simulink model "Ballbeam2020a"  (R2020a)
settings: Solver=VariableStepAuto  StartTime=0.0  StopTime=inf  RelTol=1e-3
values from neighbouring files (symbols this model uses):
  d = 0.03    [ballbeam.m]
  Den = [1 0 0]    [ballbeam.m]
  Kd = 40    [ballbeam.m]
  Kp = 15    [ballbeam.m]
  L = 1.0    (= 1)    [ballbeam.m]
  Num = [-K]    [ballbeam.m]
  R = 5    [ballbeam.m]
libraries: aerolibconvert2 x1, simulink x1, vrlib x1
settings Model: Creator=asus  LastModifiedBy=asus

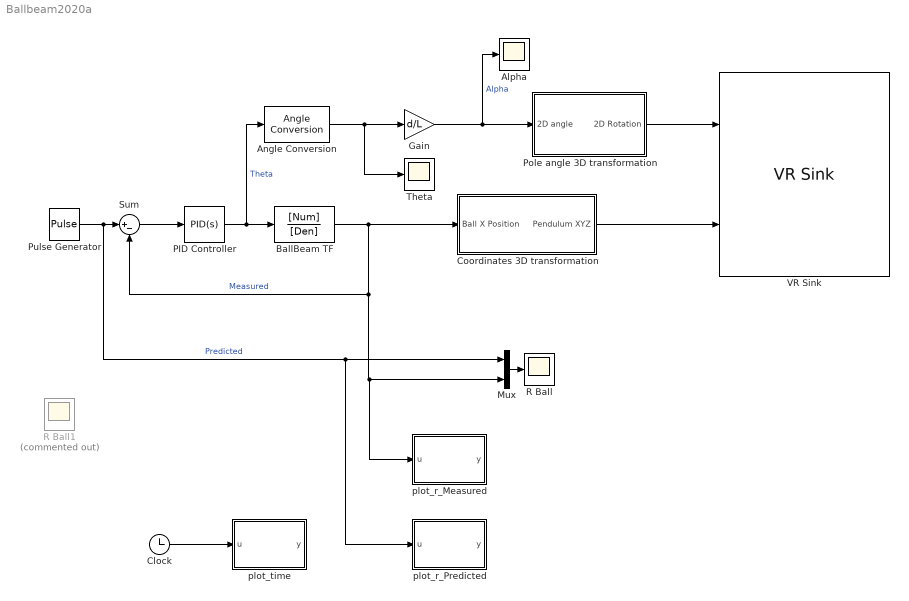
== system Ballbeam2020a ==
  "Alpha " : Scope
  Angle Conversion : aerolibconvert2/Angle Conversion  IU=deg  OU=rad
  BallBeam TF : TransferFcn  Numerator=[Num]  Denominator=[Den]
  Clock : Clock
  Coordinates 3D transformation : Subsystem
  Gain : Gain  Gain=d/L
  Mux : Mux  Inputs=2
  PID Controller : simulink/Continuous/PID Controller  Controller=PID  Form=Parallel  TimeDomain=Continuous-time  UseExternalTs=off  SampleTime=-1  IntegratorMethod=Forward Euler  FilterMethod=Forward Euler  ControllerParametersSource=internal  P=Kp  I=0  D=Kd  UseFilter=on  N=100  TunerSelectOption=Transfer Function Based (PID Tuner App)  InitialConditionSource=internal  InitialConditionForIntegrator=0  InitialConditionForFilter=0  DifferentiatorICPrevScaledInput=0  ExternalReset=none  TrackingMode=off  Kt=1  LimitOutput=off  UpperSaturationLimit=inf  LowerSaturationLimit=-inf  LinearizeAsGain=on  AntiWindupMode=none  Kb=1  POutMin=[]  POutMax=[]  IOutMin=[]  IOutMax=[]  DOutMin=[]  DOutMax=[]  NOutMin=[]  NOutMax=[]  SumOutMin=[]  SumOutMax=[]  SaturationOutMin=[]  SaturationOutMax=[]  PParamMin=[]  PParamMax=[]  IParamMin=[]  IParamMax=[]  DParamMin=[]  DParamMax=[]  NParamMin=[]  NParamMax=[]  KbParamMin=[]  KbParamMax=[]  KtParamMin=[]  KtParamMax=[]  KbOutMin=[]  KbOutMax=[]  KtOutMin=[]  KtOutMax=[]  IntegratorOutMin=[]  IntegratorOutMax=[]  FilterOutMin=[]  FilterOutMax=[]  SumI1OutMin=[]  SumI1OutMax=[]  SumI2OutMin=[]  SumI2OutMax=[]  SumI3OutMin=[]  SumI3OutMax=[]  SumI4OutMin=[]  SumI4OutMax=[]  SumDOutMin=[]  SumDOutMax=[]  DifferentiatorOutMin=[]  DifferentiatorOutMax=[]  FilterDiffOutCoefMin=[]  FilterDiffOutCoefMax=[]  ReciprocalOutMin=[]  ReciprocalOutMax=[]  SumDenOutMin=[]  SumDenOutMax=[]  SumNumOutMin=[]  SumNumOutMax=[]  DivideOutMin=[]  DivideOutMax=[]  UdiffTsProdOutMin=[]  UdiffTsProdOutMax=[]  NTsProdOutMin=[]  NTsProdOutMax=[]  UintegralTsProdOutMin=[]  UintegralTsProdOutMax=[]  UngainTsProdOutMin=[]  UngainTsProdOutMax=[]  IntegratorContinuousStateAttributes=''  IntegratorStateMustResolveToSignalObject=off  IntegratorRTWStateStorageClass=Auto  FilterContinuousStateAttributes=''  FilterStateMustResolveToSignalObject=off  FilterRTWStateStorageClass=Auto  ParallelPVariant=InternalParameters  IdealPVariant=Disabled  IVariant=InternalParameters  DVariant=InternalParameters  IntegratorVariant=Continuous  SatVariant=Disabled  AWVariant=Passthrough  PCopyVariant=Disabled  TRVariant=Disabled  FdbkBlocksVariant=Forward  IdealPFdbkVariant=Disabled  SatFdbkVariant=Disabled  DerivativeFilterVariant=ContFilter  NVariant=InternalParameters  NCopyVariant=Disabled  FilterICVariant=InternalICsFilter  IntegratorICVariant=InternalICs  ExternalResetVariant=Disabled  TRSumVariant=Passthrough  SumFdbkVariant=Disabled  SumVariant=Sum_PID  TsampFilterVariant=InternalTs  TsampNgainVariant=Passthrough  TsampIntegralVariant=Passthrough
  Pole angle 3D transformation : Subsystem
  Pulse Generator : DiscretePulseGenerator  PulseType=Time based  Amplitude=R  Period=10  PulseWidth=50
  R Ball : Scope
  R Ball1 : Scope  Commented=on
  Sum : Sum  Inputs=|+-
  Theta : Scope
  VR Sink : vrlib/VR Sink  InstantiateOnLoad=on  SampleTime=0.1  ViewEnable=on  RemoteChange=off  RemoteView=off  FieldsWritten=Batang.rotation.4.1.1.double#Bola.translation.3.1.1.double  WorldFileName=ballbeam.wrl  AutoView=off  VideoDimensions=[]  AllowVariableSize=off
  plot_r_Measured : MATLAB Function  TreatAsAtomicUnit=on
  plot_r_Predicted : MATLAB Function  TreatAsAtomicUnit=on
  plot_time : MATLAB Function  TreatAsAtomicUnit=on
  wires:
  Gain/1 -> "Alpha "/1, Pole angle 3D transformation/1(2D angle)  "Alpha"
  Mux/1 -> R Ball/1
  PID Controller/1 -> Angle Conversion/1, BallBeam TF/1  "Theta"
  Sum/1 -> PID Controller/1
  BallBeam TF/1 -> Coordinates 3D transformation/1(Ball X Position), Sum/2, plot_r_Measured/1(u), Mux/2  "Measured"
  Pulse Generator/1 -> plot_r_Predicted/1(u), Mux/1, Sum/1  "Predicted"
  Angle Conversion/1 -> Theta/1, Gain/1
  Coordinates 3D transformation/1(Pendulum XYZ) -> VR Sink/2
  Pole angle 3D transformation/1(2D Rotation) -> VR Sink/1
  Clock/1 -> plot_time/1(u)

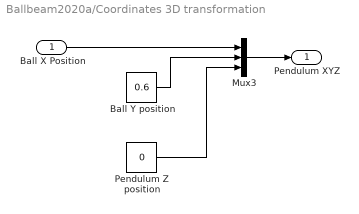
== system Ballbeam2020a/Coordinates 3D transformation ==
  Ball X Position : Inport
  Ball Y position : Constant  Value=0.6
  Mux3 : Mux  Inputs=3
  Pendulum Z position : Constant  Value=0
  Pendulum XYZ : Outport
  wires:
  Ball Y position/1 -> Mux3/2
  Mux3/1 -> Pendulum XYZ/1
  Ball X Position/1 -> Mux3/1
  Pendulum Z position/1 -> Mux3/3

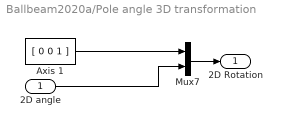
== system Ballbeam2020a/Pole angle 3D transformation ==
  2D angle : Inport
  Axis 1 : Constant  Value=[ 0 0 1 ]
  Mux7 : Mux  Inputs=2
  2D Rotation : Outport
  wires:
  Axis 1/1 -> Mux7/1
  Mux7/1 -> 2D Rotation/1
  2D angle/1 -> Mux7/2

== matlab function Ballbeam2020a/plot_time ==
  data: u input; y output
function y = run_time(u)

y = u;

== matlab function Ballbeam2020a/plot_r_Predicted ==
  data: u input; y output
function y = plot_predicted(u)

y = u;

== matlab function Ballbeam2020a/plot_r_Measured ==
  data: u input; y output
function y = plot_measured(u)

y = u;
